simulink subsystem "fix_sim"  (R2021b)
settings: Solver=FixedStepDiscrete  StartTime=0.0  StopTime=10.0  RelTol=1e-3
model mask{kernel=kernel, image_width=kernel}
  mask prompts: image_width "Image width"
settings Model: DataTypeOverride=Off  Creator=torha  LastModifiedBy=torha
settings OptimizationCC: BlockReduction=off  ConditionallyExecuteInputs=off  DefaultParameterBehavior=Inlined  InheritOutputTypeSmallerThanSingle=on
settings DebuggingCC: AlgebraicLoopMsg=error  SingleTaskRateTransMsg=error
settings HardwareCC: ProdBitPerPointer=32  ProdBitPerSizeT=32  ProdBitPerPtrDiffT=32  ProdLargestAtomicFloat=None  ProdIntDivRoundTo=Undefined  ProdEndianess=Unspecified  ProdWordSize=32  ProdHWDeviceType=ASIC/FPGA->ASIC/FPGA  TargetBitPerPointer=64  TargetBitPerSizeT=64  TargetBitPerPtrDiffT=64  TargetLongLongMode=on  TargetIntDivRoundTo=Zero  TargetEndianess=LittleEndian  TargetWordSize=64  TargetHWDeviceType=Custom Processor->MATLAB Host Computer  ProdEqTarget=off

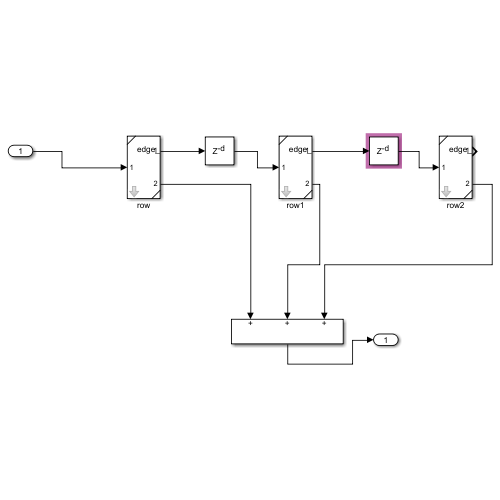
[thumbnail: Simulink's stored preview of the top-level diagram]
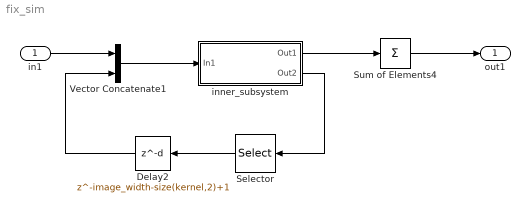
== system fix_sim ==
  in1 : Inport
  Delay2 : Delay  DelayLength=image_width-size(kernel,2)+1  InitialCondition=0
  Selector : Selector  InputPortWidth=size(kernel,1)  IndexOptions=Index vector (dialog)  Indices=1:size(kernel,1)-1  OutputSizes=1
  Sum of Elements4 : Sum  Inputs=+
  Vector Concatenate1 : Concatenate
  inner_subsystem : Subsystem  mask{kernel_rows=flip(kernel), kernel_width=size(kernel,2)}
      mask prompts: kernel_rows "Kernel"; kernel_width "Kernel width"
  out1 : Outport  VectorParamsAs1DForOutWhenUnconnected=off
  wires:
  Vector Concatenate1/1 -> inner_subsystem/1(In1)
  inner_subsystem/1(Out1) -> Sum of Elements4/1
  Selector/1 -> Delay2/1
  Delay2/1 -> Vector Concatenate1/2
  in1/1 -> Vector Concatenate1/1
  Sum of Elements4/1 -> out1/1
  inner_subsystem/2(Out2) -> Selector/1

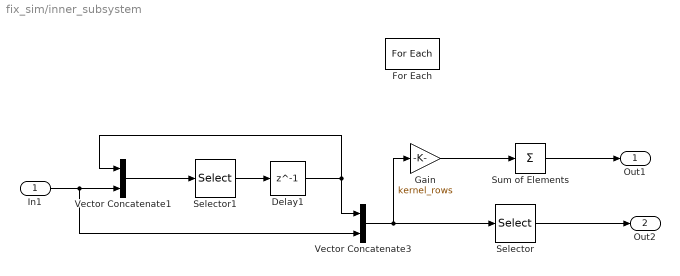
== system fix_sim/inner_subsystem ==
  In1 : Inport  PortDimensions=1  Partition=on  PartitionDimension=1  PartitionWidth=1  PartitionOffset=0
  Delay1 : Delay  DelayLength=1  InitialCondition=0
  For Each : ForEach  DisableCoverage=on  IterateSubsysMaskParameter=on,off  SubsysMaskParameterIterationDimension=1,1  SubsysMaskParameterIterationStepSize=1,1
  Gain : Gain  Gain=kernel_rows  ParamMin=-1  ParamMax=1  ParamDataTypeStr=fixdt(1,2,0)  OutDataTypeStr=fixdt(1,9,0)
  Selector : Selector  InputPortWidth=kernel_width  IndexOptions=Index vector (dialog)  Indices=1  OutputSizes=1
  Selector1 : Selector  InputPortWidth=kernel_width  IndexOptions=Index vector (dialog)  Indices=2:kernel_width  OutputSizes=1
  Sum of Elements : Sum  Inputs=+
  Vector Concatenate1 : Concatenate
  Vector Concatenate3 : Concatenate
  Out1 : Outport  ConcatenationDimension=1
  Out2 : Outport  Port=2  ConcatenationDimension=1
  wires:
  Delay1/1 -> Vector Concatenate3/1, Vector Concatenate1/1
  Selector1/1 -> Delay1/1
  Vector Concatenate1/1 -> Selector1/1
  Vector Concatenate3/1 -> Selector/1, Gain/1
  In1/1 -> Vector Concatenate1/2, Vector Concatenate3/2
  Sum of Elements/1 -> Out1/1
  Gain/1 -> Sum of Elements/1
  Selector/1 -> Out2/1
